simulink model "two_cars_with_radar"  (R2022b)
settings: Solver=VariableStepAuto  StartTime=0.0  StopTime=240  RelTol=1e-2
model workspace (MAT data in the model file):
  firstWarning = 0
  originalScenarioChecksum = 'D85659132848AD3D9BD7C7E90242BB51'
values from neighbouring files (symbols this model uses):
  b = 50    [Workspace.mat]    (also in example.mat = [65 1]; init.m; sim_params.mat)
  m = 1000    [Workspace.mat]    (also in example.mat; init.m; sim_params.mat)
  max_motor_force = 15000    [Workspace.mat]    (also in init.m; sim_params.mat = 5000)
  sign_max_break_force = -30000    [Workspace.mat]    (also in init.m)
  Ts = 0.05    [Workspace.mat]    (also in init.m; sim_params.mat = 0.1)
undefined symbols (not defined in the file or in its folder): angular, linear
libraries: simulink x4, ros2lib x2, drivingscenarioandsensors x2
settings Model: Creator=svanc  LastModifiedBy=126893
settings SolverCC: ZeroCrossControl=DisableAll  AlgebraicLoopSolver=TrustRegion
settings DebuggingCC: UnconnectedInputMsg=warning  UnconnectedOutputMsg=warning  UnconnectedLineMsg=warning  SFMachineParentedDataDiag=warning
settings ModelReferenceCC: EnableRefExpFcnMdlSchedulingChecks=on

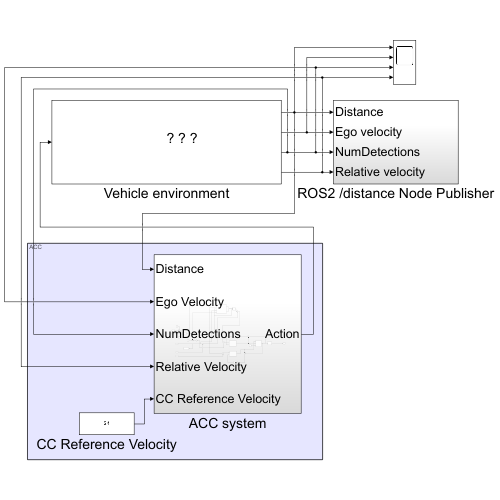
[thumbnail: Simulink's stored preview of the top-level diagram]
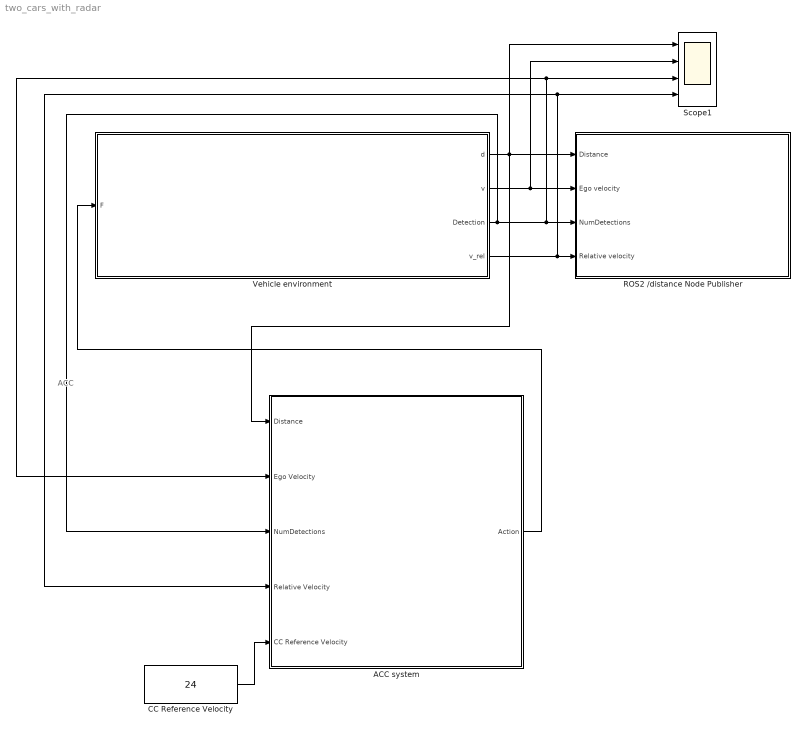
== system two_cars_with_radar ==
  note: ACC
  ACC system : Subsystem
  CC Reference Velocity : Constant  Value=24  SampleTime=Ts
  ROS2 /distance Node Publisher : Subsystem
  Scope1 : Scope  NumInputPorts=4
  Vehicle environment : Subsystem
      mask Display: image('D:\Matlab - work\BACHELOR_PROJECT\pictures\vehicle.png'); % Use "Edit Image" on toolstrip to change.
  wires:
  Vehicle environment/1(d) -> ACC system/1(Distance), ROS2 /distance Node Publisher/1(Distance), Scope1/1
  CC Reference Velocity/1 -> ACC system/5(CC Reference Velocity)
  Vehicle environment/3(Detection) -> ACC system/2(Ego Velocity), Scope1/3, ROS2 /distance Node Publisher/3(NumDetections), ACC system/3(NumDetections)
  Vehicle environment/4(v_rel) -> ACC system/4(Relative Velocity), Scope1/4, ROS2 /distance Node Publisher/4(Relative velocity)
  ACC system/1(Action) -> Vehicle environment/1("F ")
  Vehicle environment/2(v) -> Scope1/2, ROS2 /distance Node Publisher/2(Ego velocity)

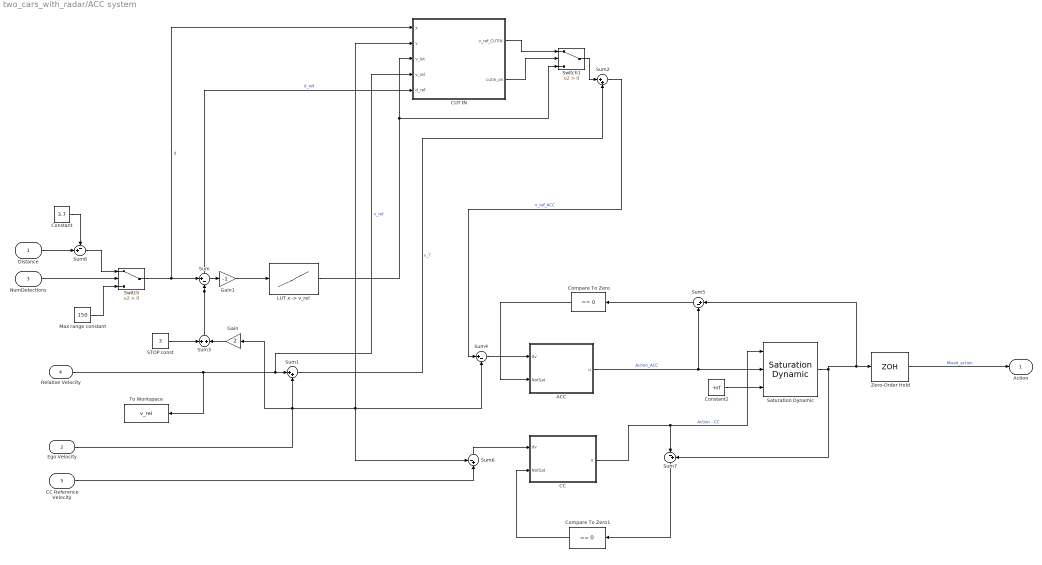
== system two_cars_with_radar/ACC system ==
  Distance : Inport
  Ego Velocity : Inport  Port=2
  NumDetections : Inport  Port=3
  Relative Velocity : Inport  Port=4
  CC Reference Velocity : Inport  Port=5
  ACC : Subsystem
  CC : Subsystem
  CUT IN : Subsystem
  Compare To Zero : simulink/Logic and Bit Operations/Compare To Zero  relop===  OutDataTypeStr=uint8
  Compare To Zero1 : simulink/Logic and Bit Operations/Compare To Zero  relop===  OutDataTypeStr=uint8
  Constant : Constant  Value=3.7
  Constant2 : Constant  Value=-inf
  Gain : Gain  Gain=2
  Gain1 : Gain  Gain=-1
  "LUT x -> v_rel" : Lookup_n-D  NumberOfTableDimensions=1  BreakpointsForDimension1=[-150;0]  Table=[0;0]  InternalRulePriority=Speed  RndMeth=Simplest
  Max range constant : Constant  Value=150  SampleTime=Ts
  STOP const : Constant  Value=3  SampleTime=Ts
  Saturation Dynamic : simulink/Discontinuities/Saturation Dynamic  OutMin=sign_max_break_force  OutMax=max_motor_force  OutDataTypeStr=Inherit: Same as second input  OutDataType=fixdt(1, 16)  OutScaling=2^-10  DoSatur=off
  Sum : Sum  Inputs=|+-
  Sum1 : Sum  Inputs=|++
  Sum2 : Sum  Inputs=|++
  Sum3 : Sum
  Sum4 : Sum  Inputs=|+-
  Sum5 : Sum  Inputs=|+-
  Sum6 : Sum  Inputs=-+|
  Sum7 : Sum  Inputs=|-+
  Sum8 : Sum  Inputs=-+|
  Switch : Switch  Criteria=u2 > Threshold  SaturateOnIntegerOverflow=off  InputSameDT=off
  Switch1 : Switch  Criteria=u2 > Threshold  SaturateOnIntegerOverflow=off  InputSameDT=off
  To Workspace : ToWorkspace  VariableName=v_rel  SampleTime=Ts
      settings: Save2DSignal=2-D array (concatenate along first dimension)
  Zero-Order Hold : ZeroOrderHold  SampleTime=Ts
  Action : Outport
  wires:
  NumDetections/1 -> Switch/2
  Max range constant/1 -> Switch/3
  Relative Velocity/1 -> To Workspace/1, CUT IN/4(v_rel), Sum1/1  "v_rel"
  Ego Velocity/1 -> Gain/1, CUT IN/2(v), Sum4/2, Sum6/1, Sum1/2
  Sum1/1 -> Sum2/2  "v_T"
  CC Reference Velocity/1 -> Sum6/2
  Sum3/1 -> CUT IN/5(d_ref), Sum/2  "d_ref"
  STOP const/1 -> Sum3/1
  Gain/1 -> Sum3/2
  Switch/1 -> Sum/1, CUT IN/1(x)  "d"
  Sum/1 -> Gain1/1
  Gain1/1 -> "LUT x -> v_rel"/1
  Sum4/1 -> ACC/1(dv)
  ACC/1(u) -> Sum5/2, Saturation Dynamic/2  "Action_ACC"
  Constant2/1 -> Saturation Dynamic/3
  Sum5/1 -> Compare To Zero/1
  Compare To Zero/1 -> ACC/2(NotSat)
  CC/1(u) -> Saturation Dynamic/1, Sum7/1  "Action - CC"
  Sum6/1 -> CC/1(dv)
  Compare To Zero1/1 -> CC/2(NotSat)
  Sum7/1 -> Compare To Zero1/1
  Distance/1 -> Sum8/2
  Constant/1 -> Sum8/1
  Sum8/1 -> Switch/1
  Saturation Dynamic/1 -> Zero-Order Hold/1, Sum5/1, Sum7/2
  Zero-Order Hold/1 -> Action/1  "Mixed_action"
  Sum2/1 -> Sum4/1  "v_ref_ACC"
  CUT IN/1(v_ref_CUTIN) -> Switch1/1
  CUT IN/2(cutin_on) -> Switch1/2
  "LUT x -> v_rel"/1 -> Switch1/3, CUT IN/3(v_lut)
  Switch1/1 -> Sum2/1

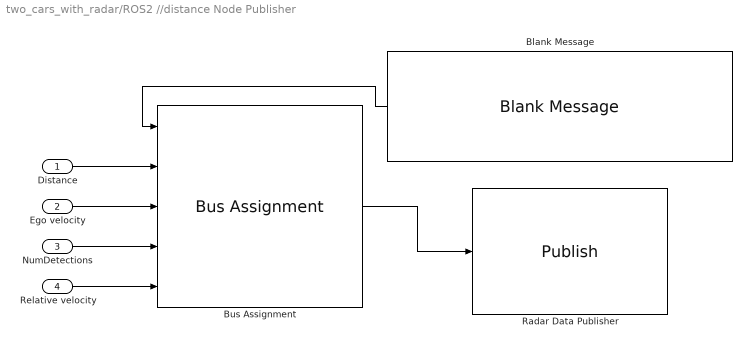
== system two_cars_with_radar/ROS2 //distance Node Publisher ==
  Distance : Inport
  Ego velocity : Inport  Port=2
  NumDetections : Inport  Port=3
  Relative velocity : Inport  Port=4
  Blank Message : ros2lib/Blank Message  messageClass=Message  entityType=geometry_msgs/Accel  messageType=geometry_msgs/Accel  SampleTime=Ts
  Bus Assignment : BusAssignment  AssignedSignals=linear.x,linear.y,linear.z,angular.x
  "Radar Data Publisher " : ros2lib/Publish  topicSource=Specify your own  topic=/distance  messageType=geometry_msgs/Accel  QOSHistory=Keep last  QOSDepth=1  QOSReliability=Reliable  QOSDurability=Volatile
  wires:
  Relative velocity/1 -> Bus Assignment/5
  Bus Assignment/1 -> "Radar Data Publisher "/1
  Blank Message/1 -> Bus Assignment/1
  Distance/1 -> Bus Assignment/2
  Ego velocity/1 -> Bus Assignment/3
  NumDetections/1 -> Bus Assignment/4

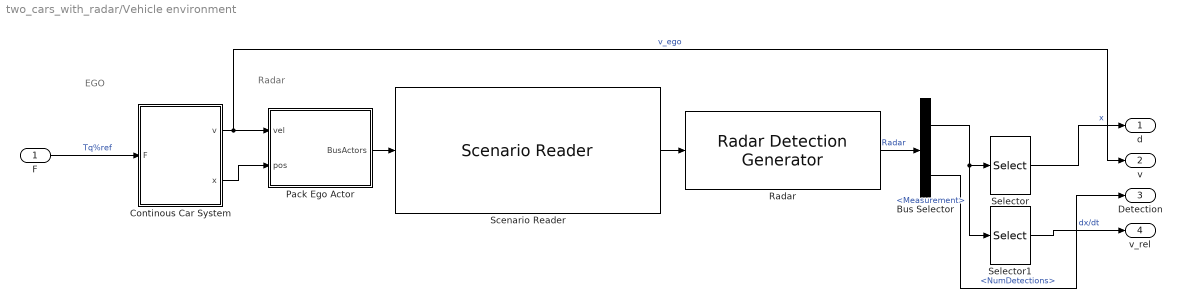
== system two_cars_with_radar/Vehicle environment ==
  note: EGO
  note: Radar
  "F " : Inport
  Bus Selector : BusSelector  OutputSignals=Detections.Measurement,NumDetections
  Continous Car System : Subsystem
  Pack Ego Actor : MATLAB Function  TreatAsAtomicUnit=on
  Radar : drivingscenarioandsensors/Radar Detection Generator  SensorIndex=1  UpdateInterval=Ts  SensorLocation=[3.7 0]  Height=0.2  Yaw=0  Pitch=0  Roll=0  BusNameSource=Auto  BusName=BusRadarDetectionGenerator  MaxNumDetectionsSource=Property  MaxNumDetections=1  DetectionCoordinates=Ego Cartesian  SimulateUsing=Interpreted execution  AzimuthResolution=4  ElevationResolution=10  RangeResolution=2.5  RangeRateResolution=0.5  AzimuthBiasFraction=0.1  ElevationBiasFraction=0.1  RangeBiasFraction=0.05  RangeRateBiasFraction=0.05  FieldOfView=[0.9 5]  MaxRange=150  RangeRateLimits=[-500 500]  DetectionProbability=1  FalseAlarmRate=1e-07  ReferenceRange=500  ReferenceRCS=0  HasElevation=off  HasRangeRate=on  HasNoise=off  HasFalseAlarms=off  HasOcclusion=off  InitialSeedSource=Repeatable  InitialSeed=0  UsedSeed=0  ActorProfilesSource=MATLAB expression  ActorProfilesParameters=driving.internal.ActorProfilesRadarParameters  ActorProfilesExpression=[struct('ActorID',1,'ClassID',1,'Length',4.7,'Width',1.8,'Height',1.4,'OriginOffset',[-1.35 0 0],'RCSPattern',[10 10;10 10],'RCSAzimuthAngles',[-180 180],'RCSElevationAngles',[-90 90]); struct('ActorID',2,'ClassID',1,'Length',4.7,'Width',1.8,'Height',1.4,'OriginOffset',[-1.35 0 0],'RCSPattern',[10 10;10 10],'RCSAzimuthAngles',[-180 180],'RCSElevationAngles',[-90 90])]
  Scenario Reader : drivingscenarioandsensors/Scenario Reader  ScenarioSource=From file  ScenarioFileName=C:\Users\126893\OneDrive-CTU\Vehicle Dynamics Control\ACC\two_cars_with_radar.mat  ScenarioVariableName=scenario  OutputCoordinateSystem=Vehicle coordinates  EgoVehicleSource=Input port  EgoVehicleActorID=1  OrientVehiclesOnRoad=off  OutputEgoVehiclePose=off  OutputEgoVehicleState=off  SampleTime=Ts  LaneBoundaryOutput=None  LaneBoundaryDistance=0:0.5:9.5  LaneBoundaryLocation=Center of lane markings  BusNameSource=Property  BusName=BusActors  BusNumActorsSource=Scenario  BusNumActors=100  BusName2Source=Auto  BusName2=BusLaneBoundaries  BusNumLaneBoundariesSource=Scenario  BusNumLaneBoundaries=10  BusName3Source=Auto  BusName3=BusEgoActor  BusName4Source=Auto  BusName4=BusEgoState  ShowCoordinateLabels=on  SimulateUsing=Interpreted execution
  Selector : Selector  InputPortWidth=6  IndexOptions=Index vector (dialog)  Indices=1  OutputSizes=1
  Selector1 : Selector  InputPortWidth=6  IndexOptions=Index vector (dialog)  Indices=4  OutputSizes=1
  d : Outport
  v : Outport  Port=2
  Detection : Outport  Port=3
  v_rel : Outport  Port=4
  wires:
  Selector1/1 -> v_rel/1  "dx/dt"
  "F "/1 -> Continous Car System/1("F ")  "Tq%ref"
  Continous Car System/2(x) -> Pack Ego Actor/2(pos)
  Bus Selector/1 -> Selector1/1, Selector/1  "<Measurement>"
  Radar/1 -> Bus Selector/1  "Radar"
  Continous Car System/1(v) -> v/1, Pack Ego Actor/1(vel)  "v_ego"
  Selector/1 -> d/1  "x"
  Pack Ego Actor/1(BusActors) -> Scenario Reader/1
  Bus Selector/2 -> Detection/1  "<NumDetections>"
  Scenario Reader/1 -> Radar/1

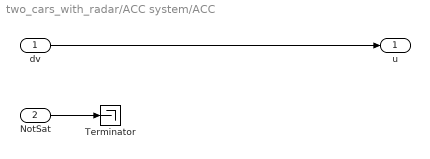
== system two_cars_with_radar/ACC system/ACC ==
  dv : Inport
  NotSat : Inport  Port=2
  Terminator : Terminator
  u : Outport
  wires:
  dv/1 -> u/1
  NotSat/1 -> Terminator/1

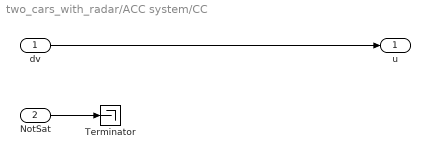
== system two_cars_with_radar/ACC system/CC ==
  dv : Inport
  NotSat : Inport  Port=2
  Terminator : Terminator
  u : Outport
  wires:
  dv/1 -> u/1
  NotSat/1 -> Terminator/1

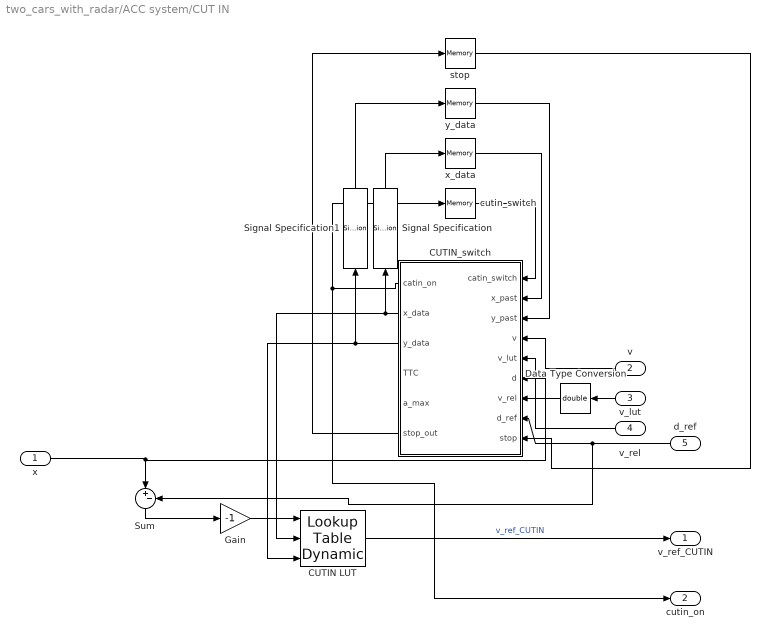
== system two_cars_with_radar/ACC system/CUT IN ==
  x : Inport
  v : Inport  Port=2
  v_lut : Inport  Port=3
  v_rel : Inport  Port=4
  d_ref : Inport  Port=5
  CUTIN LUT : simulink/Lookup Tables/Lookup Table Dynamic  LookUpMeth=Interpolation-Extrapolation  OutDataType=fixdt('double')  OutScaling=[]  OutputDataTypeScalingMode=Specify via dialog  OutDataTypeStr=double  DoSatur=off
  CUTIN_switch : MATLAB Function  TreatAsAtomicUnit=on
  Data Type Conversion : DataTypeConversion  OutDataTypeStr=double  SaturateOnIntegerOverflow=off  RndMeth=Floor
  Gain : Gain  Gain=-1
  Signal Specification : SignalSpecification  Dimensions=2  SampleTime=Ts
  Signal Specification1 : SignalSpecification  Dimensions=2  SampleTime=Ts
  Sum : Sum  Inputs=|+-
  cutin_switch : Memory
  "stop " : Memory
  x_data : Memory  InitialCondition=[-1;0]
  y_data : Memory  InitialCondition=[0;0]
  v_ref_CUTIN : Outport
  cutin_on : Outport  Port=2
  wires:
  CUTIN LUT/1 -> v_ref_CUTIN/1  "v_ref_CUTIN"
  Data Type Conversion/1 -> CUTIN_switch/5(v_lut)
  y_data/1 -> CUTIN_switch/3(y_past)
  x_data/1 -> CUTIN_switch/2(x_past)
  cutin_switch/1 -> CUTIN_switch/1(catin_switch)
  CUTIN_switch/1(catin_on) -> cutin_on/1, cutin_switch/1
  CUTIN_switch/2(x_data) -> CUTIN LUT/2, Signal Specification/1
  CUTIN_switch/3(y_data) -> CUTIN LUT/3, Signal Specification1/1
  v_lut/1 -> Data Type Conversion/1
  v/1 -> CUTIN_switch/4(v)
  v_rel/1 -> CUTIN_switch/7(v_rel)
  d_ref/1 -> Sum/2, CUTIN_switch/8(d_ref)
  Gain/1 -> CUTIN LUT/1
  x/1 -> CUTIN_switch/6(d), Sum/1
  Sum/1 -> Gain/1
  Signal Specification/1 -> x_data/1
  Signal Specification1/1 -> y_data/1
  CUTIN_switch/6(stop_out) -> "stop "/1
  "stop "/1 -> CUTIN_switch/9(stop)

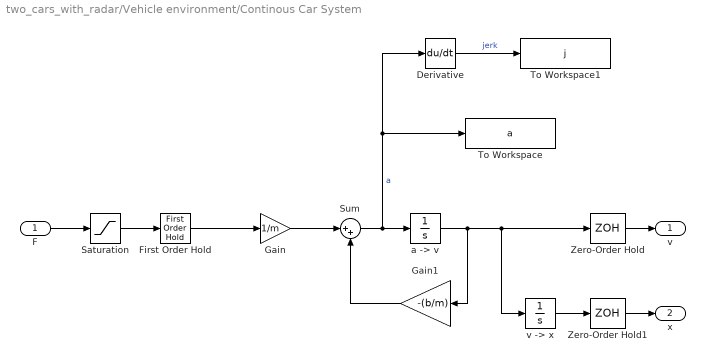
== system two_cars_with_radar/Vehicle environment/Continous Car System ==
  "F " : Inport
  Derivative : Derivative
  First Order Hold : FirstOrderHold  ErrorTolerance=inf  AllowContinuousInput=on
  Gain : Gain  Gain=1/m
  Gain1 : Gain  Gain=-(b/m)
  Saturation : Saturate  UpperLimit=max_motor_force  LowerLimit=sign_max_break_force
  Sum : Sum  Inputs=|++
  To Workspace : ToWorkspace  VariableName=a  SaveFormat=Timeseries  SampleTime=Ts
  To Workspace1 : ToWorkspace  VariableName=j  SaveFormat=Timeseries  SampleTime=Ts
  Zero-Order Hold : ZeroOrderHold  SampleTime=Ts
  Zero-Order Hold1 : ZeroOrderHold  SampleTime=Ts
  "a -> v" : Integrator  InitialCondition=23
  "v -> x" : Integrator
  v : Outport
  x : Outport  Port=2
  wires:
  "v -> x"/1 -> Zero-Order Hold1/1
  Sum/1 -> Derivative/1, To Workspace/1, "a -> v"/1  "a"
  Gain/1 -> Sum/1
  "a -> v"/1 -> Gain1/1, Zero-Order Hold/1, "v -> x"/1
  Gain1/1 -> Sum/2
  First Order Hold/1 -> Gain/1
  Zero-Order Hold/1 -> v/1
  Zero-Order Hold1/1 -> x/1
  "F "/1 -> Saturation/1
  Saturation/1 -> First Order Hold/1
  Derivative/1 -> To Workspace1/1  "jerk"

== matlab function two_cars_with_radar/ACC system/CUT IN/CUTIN_switch ==
  data: catin_switch input; catin_on output; x_past input; y_past input; v input; v_lut input; d input; x_data output; y_data output; v_rel input; TTC output; d_ref input; a_max output; stop input; stop_out output
function [catin_on, x_data, y_data, TTC, a_max, stop_out] = CUTIN_switch(catin_switch, x_past, y_past, v, v_lut, d, v_rel, d_ref, stop)
    threshold = 3;
    catin_on = catin_switch;
    
    x_data = x_past;
    y_data = y_past;
    
    delta_v = -v_rel - v_lut;
    
%     disp('x_data')
%     disp(x_data(1))
%     disp('y_data')
%     disp(y_data(1))
    d_int = d - d_ref;
%    disp(v_rel)
    TTC = d/v_rel;
    a_max = v_rel/TTC;
    stop_out = stop;
    
    
    if(catin_on ~= 1)
        if(delta_v > threshold)
            catin_on = 1;
            if(d_int > 0)
                x_data = [-d_int; 0];
                y_data = [-v_rel; 0];
            else
                x_data = [0; -d_int];
                y_data = [0; v_rel];
            end
            
                
        else
            catin_on = 0;
        end
    else
        if((v_rel >= -0.01 && v_rel <= 0.01))
            stop_out = stop + 1;
            if(stop_out > 50)
                catin_on = 0;
                stop_out = 0;
            end
        else
            stop_out = 0;
            
        end
    end
    


end

== matlab function two_cars_with_radar/Vehicle environment/Pack Ego Actor ==
  data: vel input; pos input; BusActors output Bus: BusActorsActors size=1
function BusActors = packEgo(vel, pos)

BusActors = struct(...
    'ActorID',1,...
    'Position', [0 pos 0], ...
    'Velocity', [0 vel 0], ...
    'Roll', 0, ...
    'Pitch', 0, ...
    'Yaw', 90, ...
    'AngularVelocity', [0 0 0]);

end
